simulink model "fir_vld_test"  (R2024b)
settings: Solver=VariableStepAuto  StartTime=0.0  StopTime=1  RelTol=1e-3
values from neighbouring files (symbols this model uses):
  fs_base = 48e3    (= 48000)    [main.m]
  lowpassFilt = design(lowpassSpec,'SystemObject',true)    [main.m]
libraries: dsphdlfiltering2 x1, dspsrcs4 x1
settings Model: Creator=31651  LastModifiedBy=31651

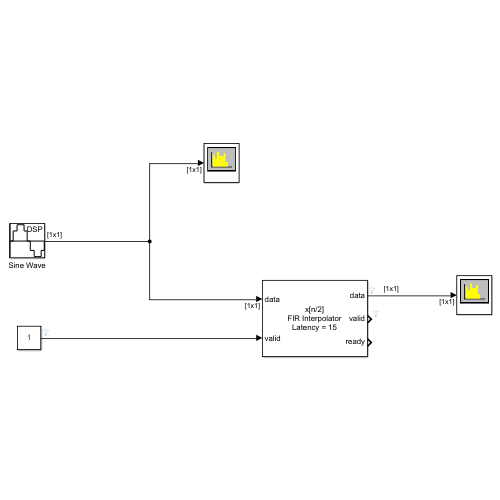
[thumbnail: Simulink's stored preview of the top-level diagram]
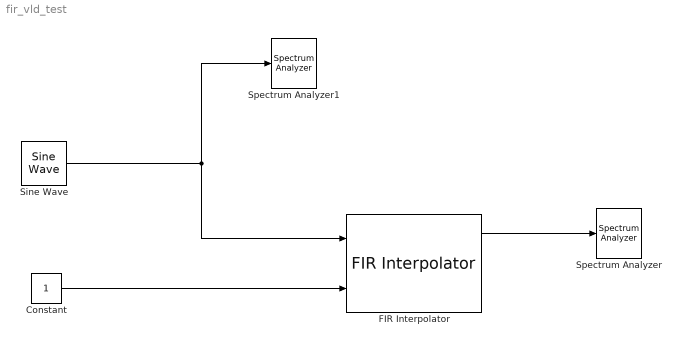
== system fir_vld_test ==
  Constant : Constant  OutDataTypeStr=boolean  SampleTime=1/fs_base
  FIR Interpolator : dsphdlfiltering2/FIR Interpolator  Numerator=lowpassFilt.Numerator  FilterStructure=Direct form systolic  InterpolationFactor=2  NumCycles=2  OptimizeSymmCoeff=on  SimulateUsing=Code generation  roundingMode=Floor  overflowMode=off  CoefficientsDataTypeStr=Inherit: Same word length as input  ResetInputPort=off  HDLGlobalReset=off
  Sine Wave : dspsrcs4/Sine Wave  Amplitude=0.9  Frequency=1000  Phase=0  SampleMode=Discrete  OutComplex=Real  CompMethod=Trigonometric fcn  TableSize=Speed  SampleTime=1/fs_base  SamplesPerFrame=1  ResetState=Restart at time zero  OutputFrames=off  dataType=double  wordLen=16  udDataType=sfix(16)  fracBitsMode=Best precision  numFracBits=15  OutDataTypeStr=double  LastOutDataTypeStr=double
  Spectrum Analyzer : SpectrumAnalyzer  WindowPosition=[880.000000,470.000000,800.000000,500.000000,]  Visible=on  ScopeFrameLocation=window  WindowInvariantSamplesPerUpdate=on  YLimits=[-67.16407782,32.57286783]
  Spectrum Analyzer1 : SpectrumAnalyzer  WindowPosition=[880.000000,470.000000,800.000000,500.000000,]  ScopeFrameLocation=window  WindowInvariantSamplesPerUpdate=on
  wires:
  Sine Wave/1 -> Spectrum Analyzer1/1, FIR Interpolator/1
  Constant/1 -> FIR Interpolator/2
  FIR Interpolator/1 -> Spectrum Analyzer/1
